simulink model "data_inspector_full_CPG"  (R2024a)
settings: Solver=ode45  StartTime=0.0  StopTime=Sim.time  MaxStep=0.00001  RelTol=1e-12  AbsTol=1e-12
settings Model: Creator=heath  LastModifiedBy=Mechatronics

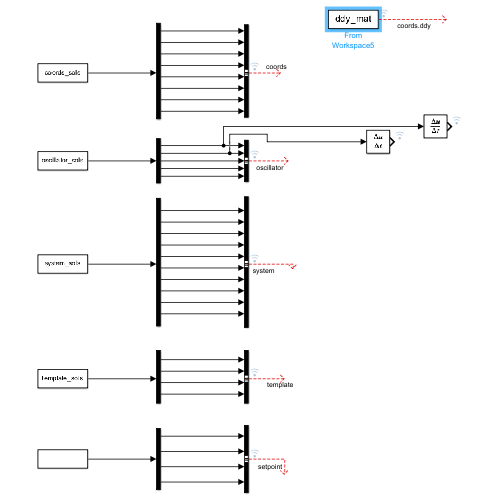
[thumbnail: Simulink's stored preview of the top-level diagram]
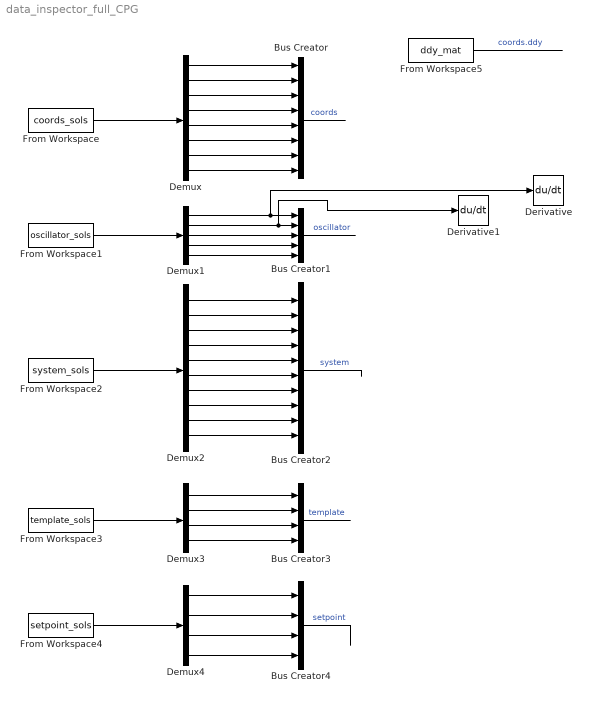
== system data_inspector_full_CPG ==
  Bus Creator : BusCreator  Inputs=8  OutDataTypeStr=Bus: Coordinate
      settings: InheritFromInputs=off
  Bus Creator1 : BusCreator  Inputs=5  OutDataTypeStr=Bus: Oscillator
      settings: InheritFromInputs=off
  Bus Creator2 : BusCreator  Inputs=10  OutDataTypeStr=Bus: System
      settings: InheritFromInputs=off
  Bus Creator3 : BusCreator  Inputs=4  OutDataTypeStr=Bus: Template
      settings: InheritFromInputs=off
  Bus Creator4 : BusCreator  Inputs=4  OutDataTypeStr=Bus: Setpoint
      settings: InheritFromInputs=off
  Demux : Demux  Outputs=8
  Demux1 : Demux  Outputs=5
  Demux2 : Demux  Outputs=10
  Demux3 : Demux
  Demux4 : Demux
  Derivative : Derivative
  Derivative1 : Derivative
  From Workspace : FromWorkspace  VariableName=coords_sols
  From Workspace1 : FromWorkspace  VariableName=oscillator_sols
  From Workspace2 : FromWorkspace  VariableName=system_sols
  From Workspace3 : FromWorkspace  VariableName=template_sols
  From Workspace4 : FromWorkspace  VariableName=setpoint_sols
  From Workspace5 : FromWorkspace  VariableName=ddy_mat
  wires:
  From Workspace2/1 -> Demux2/1
  From Workspace1/1 -> Demux1/1
  From Workspace3/1 -> Demux3/1
  Bus Creator/1 -> ?  "coords"
  Demux/8 -> Bus Creator/8
  Demux/7 -> Bus Creator/7
  Demux/6 -> Bus Creator/6
  Demux/5 -> Bus Creator/5
  Demux/4 -> Bus Creator/4
  Demux/3 -> Bus Creator/3
  Demux/2 -> Bus Creator/2
  Demux/1 -> Bus Creator/1
  From Workspace/1 -> Demux/1
  Demux1/1 -> Derivative/1, Bus Creator1/1
  Demux1/2 -> Derivative1/1, Bus Creator1/2
  Demux1/3 -> Bus Creator1/3
  Bus Creator1/1 -> ?  "oscillator"
  Bus Creator2/1 -> ?  "system"
  Demux3/1 -> Bus Creator3/1
  Demux3/2 -> Bus Creator3/2
  Demux3/3 -> Bus Creator3/3
  Demux3/4 -> Bus Creator3/4
  Bus Creator3/1 -> ?  "template"
  From Workspace4/1 -> Demux4/1
  Demux4/2 -> Bus Creator4/2
  Demux4/1 -> Bus Creator4/1
  Demux4/3 -> Bus Creator4/3
  Bus Creator4/1 -> ?  "setpoint"
  Demux2/8 -> Bus Creator2/8
  Demux2/7 -> Bus Creator2/7
  Demux2/6 -> Bus Creator2/6
  Demux2/5 -> Bus Creator2/5
  Demux2/4 -> Bus Creator2/4
  Demux2/3 -> Bus Creator2/3
  Demux2/2 -> Bus Creator2/2
  Demux2/1 -> Bus Creator2/1
  Demux2/9 -> Bus Creator2/9
  Demux2/10 -> Bus Creator2/10
  Demux1/4 -> Bus Creator1/4
  Demux1/5 -> Bus Creator1/5
  Demux4/4 -> Bus Creator4/4
  From Workspace5/1 -> ?  "coords.ddy"
